simulink model "VCU_SW_1"  (R2023b)
settings: Solver=FixedStepDiscrete  StartTime=0.0  StopTime=inf  FixedStep=1e-2  RelTol=1e-3
PreLoadFcn:
  | RTWConfigurationCB('preloadfcn', bdroot);
InitFcn:
  | loadvar_ttc500
undefined symbols (not defined in the file): BrkPedalTypes, CabMovModeTypes, cFuseTempSensAcc_X, cFuseTempSensAcc_Y, cFuseTempSensVal_X, cFuseTempSensVal_Y, cTMSTempSensVal_X, cTMSTempSensVal_Y, cTransferCaseSpeedRatio, diag_state, DoorsPositionTypes, dP_filter_Y, DriverOccClassSystemTypes, ErrorValueTypes, fatal_error_callback, IO_ADC_NO_RANGE, LadderStatusTypes, pAnalogCabRotSensAcc, pAnalogCabRotSensMaxVolt, pAnalogCabRotSensMinVolt, pAnalogCabRotSensRange, pAnalogCabRotSensZeroVolt, pBrkActivePress, pCabTiltSensAcc, pCabTiltSensMaxCur, pCabTiltSensMinCur, pDistanceCorrection, pECANManual_BPNEnable, pECANManual_BPNEnabler_Flag, pFilterSensAccRes, pHDirMaxDiffFrq, pHDirSensHighLvl, pHDirSensLowLvl, pMainGearRatio, pMaxFilterSensRes, pMaxFirstPedalSensValue, pMaxFuseTempSensRes, pMaxPressLoss, pMaxPressSensCurrent, pMaxPressValue, pMaxPressValueHydMotAndPump, pMaxPressValueParkDrain, pMaxSecondPedalSensValue, pMaxTempSensVoltage, pMaxTempValue, pMaxTMSTempSensRes, pMinFilterSensRes, pMinFirstPedalSensValue, pMinFuseTempSensRes, pMinPressLoss, pMinPressSensCurrent, pMinPressValue, pMinSecondPedalSensValue, pMinTempSensVoltage, pMinTempValue, pMinTMSTempSensRes, pMotorRingTeethNum, pPedalSensAccuracyPct, pPedalSensAccuracyVolt, pPressLossTreshhold ... (+20)
libraries: TTlibrary x270, canmsglib x127, simulink x88
(part 6 of 19)

== system VCU_SW_1/InputLayer/Manual/GetManual/TSC1 ==
  CAN_ManualData_TSC1 : canmsglib/CAN Unpack  MsgList=(none)  MsgName=Man_TSC1  MsgIDType=Extended (29-bit identifier)  MsgIdentifier=402659111  MsgLength=8  SignalInfo={ 'Man_ContPurp', '35', '5', 'LE', 'unsigned', 'Standard', '0', '1', '0', '0', '31'; 'Man_EngOverContMode', '27', '2', 'LE', 'unsigned', 'Standard', '0', '1', '0', '0', '3'; 'Man_EngReqSpSl', '8', '16', 'LE', 'unsigned', 'Standard', '0', '0.125', '0', '0', '8191.875'; 'Man_EngReqTrqTL', '0', '8', 'LE', 'unsigned', 'Standard', '0', '1', '-125', '-125', '130'; 'Man_F_ContPurp', '40', '1', 'LE', 'unsigned', 'Standard', '0', '1', '0', '0', '1'; 'Man_F_EngOverContMode', '29', '1', 'LE', 'unsigned', 'Standard', '0', '1', '0', '0', '1'; 'Man_F_EngReqSpSl', '31', '1', 'LE', 'unsigned', 'Standard', '0', '1', '0', '0', '1'; 'Man_F_EngReqTrqTL', '30', '1', 'LE', 'unsigned', 'Standard', '0', '1', '0', '0', '1'; 'Man_F_OverContModePr', '34', '1', 'LE', 'unsigned', 'Standard', '0', '1', '0', '0', '1'; 'Man_F_ReqSpContCond', '26', '1', 'LE', 'unsigned', 'Standard', '0', '1', '0', '0', '1'; 'Man_OverContModePr', '32', '2', 'LE', 'unsigned', 'Standard', '0', '1', '0', '0', '3'; 'Man_ReqSpContCond', '24', '2', 'LE', 'unsigned', 'Standard', '0', '1', '0', '0', '3' }  IDPort=off  TimestampPort=off  ErrorPort=off  RemotePort=off  LengthPort=off  StatusPort=off  ApplyMinMax=off
  Data Store Write1 : DataStoreWrite  DataStoreName=ManualOutputInterfaceData  DataStoreElements=ManualOutputInterfaceData.TSC1_Man.Man_ContPurp#ManualOutputInterfaceData.TSC1_Man.Man_EngOverContMode#ManualOutputInterfaceData.TSC1_Man.Man_EngReqSpSl#ManualOutputInterfaceData.TSC1_Man.Man_EngReqTrqTL#ManualOutputInterfaceData.TSC1_Man.Man_F_ContPurp#ManualOutputInterfaceData.TSC1_Man.Man_F_EngOverContMode#ManualOutputInterfaceData.TSC1_Man.Man_F_EngReqSpSl#ManualOutputInterfaceData.TSC1_Man.Man_F_EngReqTrqTL#ManualOutputInterfaceData.TSC1_Man.Man_F_OverContModePr#ManualOutputInterfaceData.TSC1_Man.Man_F_ReqSpContCond#ManualOutputInterfaceData.TSC1_Man.Man_OverContModePr#ManualOutputInterfaceData.TSC1_Man.Man_ReqSpContCond  IndexOptions=Index vector (dialog)  Indices=1  OutputSizes=1
  Data Type Conversion : DataTypeConversion  OutDataTypeStr=int8  SaturateOnIntegerOverflow=off  RndMeth=Floor
  Terminator1 : Terminator
  read_message_ManualData_TSC1 : TTlibrary/CAN/read_message_name  channel=IO_CAN_CHANNEL_6  id_format=IO_CAN_EXT_FRAME  get_msg_info=off  message_names=there is no CAN Unpack blocks  message_info=|  id=402659111  ac_mask=536870911  retranslation=off  io_error=on  sample_time=-1
      | Message Name: Man_TSC1
      |  Message ID Type: Extended (29-bit identifier)
      |  Message ID: 402659111
      settings: SourceProductName=TT control 500 series
  wires:
  Data Type Conversion/1 -> Data Store Write1/4
  CAN_ManualData_TSC1/12 -> Data Store Write1/12
  CAN_ManualData_TSC1/11 -> Data Store Write1/11
  CAN_ManualData_TSC1/10 -> Data Store Write1/10
  CAN_ManualData_TSC1/9 -> Data Store Write1/9
  CAN_ManualData_TSC1/8 -> Data Store Write1/8
  CAN_ManualData_TSC1/7 -> Data Store Write1/7
  CAN_ManualData_TSC1/6 -> Data Store Write1/6
  CAN_ManualData_TSC1/5 -> Data Store Write1/5
  CAN_ManualData_TSC1/4 -> Data Type Conversion/1
  CAN_ManualData_TSC1/3 -> Data Store Write1/3
  CAN_ManualData_TSC1/2 -> Data Store Write1/2
  CAN_ManualData_TSC1/1 -> Data Store Write1/1
  read_message_ManualData_TSC1/2 -> Terminator1/1  "handler_err_402659111"
  read_message_ManualData_TSC1/1 -> CAN_ManualData_TSC1/1  "msg_402659111"

== system VCU_SW_1/InputLayer/Manual/GetManual/VLVCMD_HYD ==
  Data Store Write3 : DataStoreWrite  DataStoreName=ManualOutputInterfaceData  DataStoreElements=ManualOutputInterfaceData.VLVCMD_HYD.Man_Cab1LeftCylPortFlowCmdHyd#ManualOutputInterfaceData.VLVCMD_HYD.Man_Cab1LeftCylValveStateHyd#ManualOutputInterfaceData.VLVCMD_HYD.Man_Cab2RightCylFailSafeModeCmdHyd#ManualOutputInterfaceData.VLVCMD_HYD.Man_Cab2RightCylPortFlowCmdHyd#ManualOutputInterfaceData.VLVCMD_HYD.Man_Cab2RightCylValveStateHyd#ManualOutputInterfaceData.VLVCMD_HYD.Man_Cab1LeftCylFailSafeModeCmdHyd#ManualOutputInterfaceData.VLVCMD_HYD.Man_CabRotFailSafeModeCmdHyd#ManualOutputInterfaceData.VLVCMD_HYD.Man_CabRotPortFlowCmdHyd#ManualOutputInterfaceData.VLVCMD_HYD.Man_CabRotValveStateHyd#ManualOutputInterfaceData.VLVCMD_HYD.Man_F_Cab1LeftCylFailSafeModeCmdHyd#ManualOutputInterfaceData.VLVCMD_HYD.Man_F_Cab1LeftCylPortFlowCmdHyd#ManualOutputInterfaceData.VLVCMD_HYD.Man_F_Cab1LeftCylValveStateHyd#ManualOutputInterfaceData.VLVCMD_HYD.Man_F_Cab2RightCylFailSafeModeCmdHyd#ManualOutputInterfaceData.VLVCMD_HYD.Man_F_Cab2RightCylPortFlowCmdHyd#ManualOutputInterfaceData.VLVCMD_HYD.Man_F_Cab2RightCylValveStateHyd#ManualOutputInterfaceData.VLVCMD_HYD.Man_F_CabRotFailSafeModeCmdHyd#ManualOutputInterfaceData.VLVCMD_HYD.Man_F_CabRotPortFlowCmdHyd#ManualOutputInterfaceData.VLVCMD_HYD.Man_F_CabRotValveStateHyd  IndexOptions=Index vector (dialog)  Indices=1  OutputSizes=1
  Man_EEC2 : canmsglib/CAN Unpack  MsgList=(none)  MsgName=Man_VLVCMD_HYD  MsgIDType=Extended (29-bit identifier)  MsgIdentifier=402659879  MsgLength=8  SignalInfo={ 'Man_Cab1LeftCylPortFlowCmdHyd', '17', '8', 'LE', 'unsigned', 'Standard', '0', '0.4', '0', '0', '100'; 'Man_Cab1LeftCylValveStateHyd', '25', '4', 'LE', 'unsigned', 'Standard', '0', '1', '0', '0', '15'; 'Man_Cab2RightCylFailSafeModeCmd', '46', '2', 'LE', 'unsigned', 'Standard', '0', '1', '0', '0', '3'; 'Man_Cab2RightCylPortFlowCmdHyd', '34', '8', 'LE', 'unsigned', 'Standard', '0', '0.4', '0', '0', '100'; 'Man_Cab2RightCylValveStateHyd', '42', '4', 'LE', 'unsigned', 'Standard', '0', '1', '0', '0', '15'; 'Man_CabLeftCylFailSafeModeCmdHyd', '29', '2', 'LE', 'unsigned', 'Standard', '0', '1', '0', '0', '3'; 'Man_CabRotFailSafeModeCmdHyd', '12', '2', 'LE', 'unsigned', 'Standard', '0', '1', '0', '0', '3'; 'Man_CabRotPortFlowCmdHyd', '0', '8', 'LE', 'unsigned', 'Standard', '0', '0.4', '0', '0', '100'; 'Man_CabRotValveStateHyd', '8', '4', 'LE', 'unsigned', 'Standard', '0', '1', '0', '0', '15'; 'Man_F_Cab1LeftCylFailSafeModeCmd', '33', '1', 'LE', 'unsigned', 'Standard', '0', '1', '0', '0', '1'; 'Man_F_Cab1LeftCylPortFlowCmd', '31', '1', 'LE', 'unsigned', 'Standard', '0', '1', '0', '0', '1'; 'Man_F_Cab1LeftCylValveState', '32', '1', 'LE', 'unsigned', 'Standard', '0', '1', '0', '0', '1'; 'Man_F_Cab2RightCylFailSafeMode', '50', '1', 'LE', 'unsigned', 'Standard', '0', '1', '0', '0', '1'; 'Man_F_Cab2RightCylPortFlowCmd', '48', '1', 'LE', 'unsigned', 'Standard', '0', '1', '0', '0', '1'; 'Man_F_Cab2RightCylValveState', '49', '1', 'LE', 'unsigned', 'Standard', '0', '1', '0', '0', '1'; 'Man_F_CabRotFailSafeModeCmdHyd', '16', '1', 'LE', 'unsigned', 'Standard', '0', '1', '0', '0', '1'; 'Man_F_CabRotPortFlowCmdHyd', '14', '1', 'LE', 'unsigned', 'Standard', '0', '1', '0', '0', '1'; 'Man_F_CabRotValveStateHyd', '15', '1', 'LE', 'unsigned', 'Standard', '0', '1', '0', '0', '1' }  IDPort=off  TimestampPort=off  ErrorPort=off  RemotePort=off  LengthPort=off  StatusPort=off  ApplyMinMax=off
  Terminator1 : Terminator
  read_message_Man_EEC2 : TTlibrary/CAN/read_message_name  channel=IO_CAN_CHANNEL_6  id_format=IO_CAN_EXT_FRAME  get_msg_info=off  message_names=there is no CAN Unpack blocks  message_info=|  id=402660135  ac_mask=536870911  retranslation=off  io_error=on  sample_time=-1
      | Message Name: Man_TSC1
      |  Message ID Type: Extended (29-bit identifier)
      |  Message ID: 402659111
      settings: SourceProductName=TT control 500 series
  wires:
  read_message_Man_EEC2/1 -> Man_EEC2/1  "msg_402660135"
  Man_EEC2/17 -> Data Store Write3/17
  Man_EEC2/18 -> Data Store Write3/18
  Man_EEC2/14 -> Data Store Write3/14
  Man_EEC2/15 -> Data Store Write3/15
  Man_EEC2/12 -> Data Store Write3/12
  Man_EEC2/13 -> Data Store Write3/13
  Man_EEC2/16 -> Data Store Write3/16
  Man_EEC2/10 -> Data Store Write3/10
  Man_EEC2/9 -> Data Store Write3/9
  Man_EEC2/6 -> Data Store Write3/6
  read_message_Man_EEC2/2 -> Terminator1/1  "handler_err_402660135"
  Man_EEC2/7 -> Data Store Write3/7
  Man_EEC2/11 -> Data Store Write3/11
  Man_EEC2/8 -> Data Store Write3/8
  Man_EEC2/4 -> Data Store Write3/4
  Man_EEC2/2 -> Data Store Write3/2
  Man_EEC2/1 -> Data Store Write3/1
  Man_EEC2/3 -> Data Store Write3/3
  Man_EEC2/5 -> Data Store Write3/5

== system VCU_SW_1/InputLayer/Manual/GetManual/VLVCMD_STR ==
  CAN_ManualData_Params1 : canmsglib/CAN Unpack  MsgList=(none)  MsgName=Man_VLVCMD_STR  MsgIDType=Extended (29-bit identifier)  MsgIdentifier=402659623  MsgLength=8  SignalInfo={ 'Man_F_FailSafeModeCmdStr', '16', '1', 'LE', 'unsigned', 'Standard', '0', '1', '0', '0', '1'; 'Man_F_PortFlowCmdStr', '14', '1', 'LE', 'unsigned', 'Standard', '0', '1', '0', '0', '1'; 'Man_F_ValveStateStr', '15', '1', 'LE', 'unsigned', 'Standard', '0', '1', '0', '0', '1'; 'Man_FailSafeModeCmdStr', '12', '2', 'LE', 'unsigned', 'Standard', '0', '1', '0', '0', '3'; 'Man_PortFlowCmdStr', '0', '8', 'LE', 'unsigned', 'Standard', '0', '0.4', '0', '0', '100'; 'Man_ValveStateStr', '8', '4', 'LE', 'unsigned', 'Standard', '0', '1', '0', '0', '15' }  IDPort=off  TimestampPort=off  ErrorPort=off  RemotePort=off  LengthPort=off  StatusPort=off  ApplyMinMax=off
  Data Store Write2 : DataStoreWrite  DataStoreName=ManualOutputInterfaceData  DataStoreElements=ManualOutputInterfaceData.VLVCMD_STR.Man_F_FailSafeModeCmdStr#ManualOutputInterfaceData.VLVCMD_STR.Man_F_PortFlowCmdStr#ManualOutputInterfaceData.VLVCMD_STR.Man_F_ValveStateStr#ManualOutputInterfaceData.VLVCMD_STR.Man_FailSafeModeCmdStr#ManualOutputInterfaceData.VLVCMD_STR.Man_PortFlowCmdStr#ManualOutputInterfaceData.VLVCMD_STR.Man_ValveStateStr  IndexOptions=Index vector (dialog)  Indices=1  OutputSizes=1
  Terminator2 : Terminator
  read_message_ManualData_Params : TTlibrary/CAN/read_message_name  channel=IO_CAN_CHANNEL_6  id_format=IO_CAN_EXT_FRAME  get_msg_info=off  message_names=there is no CAN Unpack blocks  message_info=|  id=402659623  ac_mask=536870911  retranslation=off  io_error=on  sample_time=-1
      | Message Name: Man_Params
      |  Message ID Type: Extended (29-bit identifier)
      |  Message ID: 402658855
      settings: SourceProductName=TT control 500 series
  wires:
  CAN_ManualData_Params1/6 -> Data Store Write2/6
  CAN_ManualData_Params1/5 -> Data Store Write2/5
  CAN_ManualData_Params1/4 -> Data Store Write2/4
  CAN_ManualData_Params1/3 -> Data Store Write2/3
  CAN_ManualData_Params1/2 -> Data Store Write2/2
  CAN_ManualData_Params1/1 -> Data Store Write2/1
  read_message_ManualData_Params/2 -> Terminator2/1  "handler_err_402659623"
  read_message_ManualData_Params/1 -> CAN_ManualData_Params1/1  "msg_402659623"

== system VCU_SW_1/OutputLayer/OutputInterfaces/DigitalOutput1/SetDO1000msec ==
  function : TriggerPort  TriggerType=function-call  VariantControl=Variant
  Constant48 : Constant  Value=2  OutDataTypeStr=uint8
  Constant49 : Constant  OutDataTypeStr=uint8
  Data Store Read15 : DataStoreRead  DataStoreName=OutputInterfaceData  DataStoreElements=OutputInterfaceData.DO.lowBrakeFluidSensSupply  IndexOptions=Index vector (dialog)  Indices=1  OutputSizes=1
  Data Store Read61 : DataStoreRead  DataStoreName=ManualOutputInterfaceData  DataStoreElements=ManualOutputInterfaceData.DO_Man.man_lowBrakeFluidSensSupply  IndexOptions=Index vector (dialog)  Indices=1  OutputSizes=1
  Data Type Conversion25 : DataTypeConversion  OutDataTypeStr=boolean  SaturateOnIntegerOverflow=off  RndMeth=Floor
  Function Caller16 : FunctionCaller  FunctionPrototype=rawValue = convDIOStsTypeToNum(enumValue)  InputArgumentSpecifications=<Enter example>  OutputArgumentSpecifications=<Enter example>
  Logical Operator25 : Logic  Operator=OR  AllPortsSameDT=off  OutDataTypeStr=boolean
  Multiport Switch25 : MultiPortSwitch  DataPortOrder=Zero-based contiguous  Inputs=2  zeroidx=on  SaturateOnIntegerOverflow=off  InputSameDT=off
  Relational Operator50 : RelationalOperator  Operator===  OutDataTypeStr=boolean  RndMeth=Simplest  InputSameDT=off
  Relational Operator51 : RelationalOperator  Operator===  OutDataTypeStr=boolean  RndMeth=Simplest  InputSameDT=off
  Subsystem : Subsystem
  Terminator10 : Terminator
  setDigitalOutputValue16 : TTlibrary/DIO/setDigitalOutputValue  do_channel=IO_DO_41  diagnostic=FALSE  safety_conf=off  low_side_safety_channel=IO_DO_08  io_error=on  sample_time=-1
      settings: SourceProductName=TT control 500 series
  wires:
  Data Type Conversion25/1 -> Multiport Switch25/3
  Constant49/1 -> Relational Operator50/2
  Relational Operator50/1 -> Logical Operator25/2
  Multiport Switch25/1 -> setDigitalOutputValue16/1
  Logical Operator25/1 -> Multiport Switch25/1
  Data Store Read15/1 -> Function Caller16/1
  Relational Operator51/1 -> Logical Operator25/1
  Data Store Read61/1 -> Relational Operator51/1, Relational Operator50/1, Subsystem/1(In1)
  setDigitalOutputValue16/1 -> Terminator10/1
  Constant48/1 -> Relational Operator51/2
  Function Caller16/1 -> Multiport Switch25/2
  Subsystem/1(Out1) -> Data Type Conversion25/1

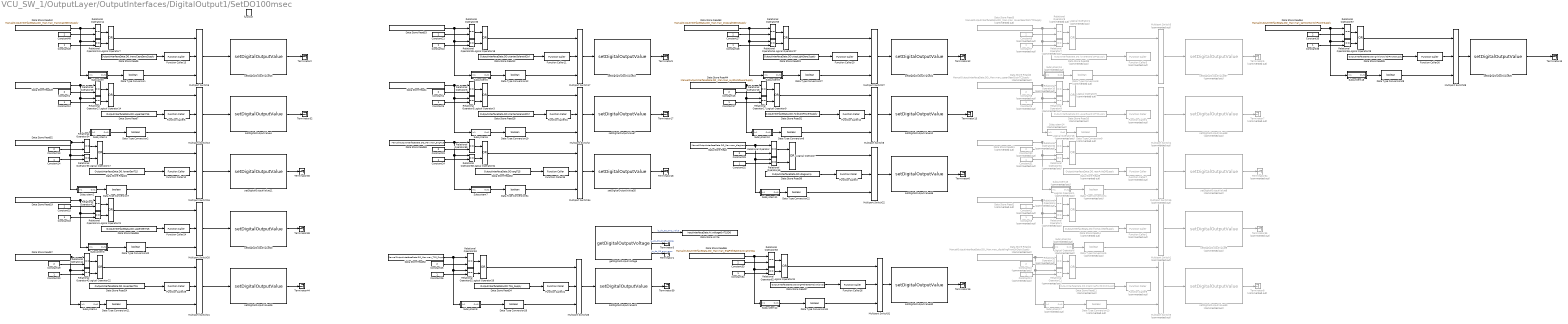
== system VCU_SW_1/OutputLayer/OutputInterfaces/DigitalOutput1/SetDO100msec ==
  function : TriggerPort  TriggerType=function-call  VariantControl=Variant
  Constant{1,4,13,15..16,19,21,23,25,27,29,33,35,48} (14 alike) : Constant  Value=2  OutDataTypeStr=uint8
  Constant{2,6,8,10,30} (5 alike) : Constant  Commented=on  Value=2  OutDataTypeStr=uint8
  Constant{3,7,9,11,31} (5 alike) : Constant  Commented=on  OutDataTypeStr=uint8
  Constant{5,12,14,17..18,20,22,24,26,28,32,34,36,49} (14 alike) : Constant  OutDataTypeStr=uint8
  Data Store Read : DataStoreRead  DataStoreName=ManualOutputInterfaceData  DataStoreElements=ManualOutputInterfaceData.DO_Man.man_diagLamp  IndexOptions=Index vector (dialog)  Indices=1  OutputSizes=1
  Data Store Read10 : DataStoreRead  Commented=on  DataStoreName=OutputInterfaceData  DataStoreElements=OutputInterfaceData.DO.upperGearDistrTCSupply  IndexOptions=Index vector (dialog)  Indices=1  OutputSizes=1
  Data Store Read11 : DataStoreRead  Commented=on  DataStoreName=OutputInterfaceData  DataStoreElements=OutputInterfaceData.DO.disablingFrontDrDistrSupply  IndexOptions=Index vector (dialog)  Indices=1  OutputSizes=1
  Data Store Read12 : DataStoreRead  DataStoreName=OutputInterfaceData  DataStoreElements=OutputInterfaceData.DO.starterSolenoidCtrl  IndexOptions=Index vector (dialog)  Indices=1  OutputSizes=1
  Data Store Read14 : DataStoreRead  Commented=on  DataStoreName=OutputInterfaceData  DataStoreElements=OutputInterfaceData.DO.frontAxleDifSupply  IndexOptions=Index vector (dialog)  Indices=1  OutputSizes=1
  Data Store Read19 : DataStoreRead  DataStoreName=ManualOutputInterfaceData  DataStoreElements=ManualOutputInterfaceData.DO_Man.man_upperGenT15  IndexOptions=Index vector (dialog)  Indices=1  OutputSizes=1
  Data Store Read2 : DataStoreRead  Commented=on  DataStoreName=ManualOutputInterfaceData  DataStoreElements=ManualOutputInterfaceData.DO_Man.man_frontAxleDifSupply  IndexOptions=Index vector (dialog)  Indices=1  OutputSizes=1
  Data Store Read22 : DataStoreRead  DataStoreName=OutputInterfaceData  DataStoreElements=OutputInterfaceData.DO.lowerGenT15  IndexOptions=Index vector (dialog)  Indices=1  OutputSizes=1
  Data Store Read23 : DataStoreRead  DataStoreName=OutputInterfaceData  DataStoreElements=OutputInterfaceData.DO.stopLightSensSupply  IndexOptions=Index vector (dialog)  Indices=1  OutputSizes=1
  Data Store Read24 : DataStoreRead  DataStoreName=OutputInterfaceData  DataStoreElements=OutputInterfaceData.DO.lowerGenT15  IndexOptions=Index vector (dialog)  Indices=1  OutputSizes=1
  Data Store Read27 : DataStoreRead  DataStoreName=OutputInterfaceData  DataStoreElements=OutputInterfaceData.DO.engPreheaterActivationSig  IndexOptions=Index vector (dialog)  Indices=1  OutputSizes=1
  Data Store Read28 : DataStoreRead  DataStoreName=OutputInterfaceData  DataStoreElements=OutputInterfaceData.DO.starterSolenoidCtrl  IndexOptions=Index vector (dialog)  Indices=1  OutputSizes=1
  Data Store Read3 : DataStoreRead  Commented=on  DataStoreName=ManualOutputInterfaceData  DataStoreElements=ManualOutputInterfaceData.DO_Man.man_lowerGearDistrTCSupply  IndexOptions=Index vector (dialog)  Indices=1  OutputSizes=1
  Data Store Read31 : DataStoreRead  DataStoreName=OutputInterfaceData  DataStoreElements=OutputInterfaceData.DO.HydCANPowerSupply  IndexOptions=Index vector (dialog)  Indices=1  OutputSizes=1
  Data Store Read32 : DataStoreRead  DataStoreName=OutputInterfaceData  DataStoreElements=OutputInterfaceData.DO.engT15  IndexOptions=Index vector (dialog)  Indices=1  OutputSizes=1
  Data Store Read34 : DataStoreRead  DataStoreName=OutputInterfaceData  DataStoreElements=OutputInterfaceData.DO.T15_Supply  IndexOptions=Index vector (dialog)  Indices=1  OutputSizes=1
  Data Store Read35 : DataStoreRead  DataStoreName=OutputInterfaceData  DataStoreElements=OutputInterfaceData.DO.IgnitionSwitchPowerSupply  IndexOptions=Index vector (dialog)  Indices=1  OutputSizes=1
  Data Store Read36 : DataStoreRead  DataStoreName=OutputInterfaceData  DataStoreElements=OutputInterfaceData.DO.diagLamp  IndexOptions=Index vector (dialog)  Indices=1  OutputSizes=1
  Data Store Read39 : DataStoreRead  Commented=on  DataStoreName=OutputInterfaceData  DataStoreElements=OutputInterfaceData.DO.lowerGearDistrTCSupply  IndexOptions=Index vector (dialog)  Indices=1  OutputSizes=1
  Data Store Read4 : DataStoreRead  DataStoreName=ManualOutputInterfaceData  DataStoreElements=ManualOutputInterfaceData.DO_Man.man_starterSolenoidCtrl  IndexOptions=Index vector (dialog)  Indices=1  OutputSizes=1
  Data Store Read40 : DataStoreRead  Commented=on  DataStoreName=ManualOutputInterfaceData  DataStoreElements=ManualOutputInterfaceData.DO_Man.man_upperGearDistrTCSupply  IndexOptions=Index vector (dialog)  Indices=1  OutputSizes=1
  Data Store Read41 : DataStoreRead  Commented=on  DataStoreName=ManualOutputInterfaceData  DataStoreElements=ManualOutputInterfaceData.DO_Man.man_disablingFrontDrDistrSupply  IndexOptions=Index vector (dialog)  Indices=1  OutputSizes=1
  Data Store Read42 : DataStoreRead  DataStoreName=ManualOutputInterfaceData  DataStoreElements=ManualOutputInterfaceData.DO_Man.man_transCaseSensSupply  IndexOptions=Index vector (dialog)  Indices=1  OutputSizes=1
  Data Store Read44 : DataStoreRead  DataStoreName=ManualOutputInterfaceData  DataStoreElements=ManualOutputInterfaceData.DO_Man.man_HydCANPowerSupply  IndexOptions=Index vector (dialog)  Indices=1  OutputSizes=1
  Data Store Read49 : DataStoreRead  DataStoreName=ManualOutputInterfaceData  DataStoreElements=ManualOutputInterfaceData.DO_Man.man_upperGenT15  IndexOptions=Index vector (dialog)  Indices=1  OutputSizes=1
  Data Store Read5 : DataStoreRead  DataStoreName=OutputInterfaceData  DataStoreElements=OutputInterfaceData.DO.transCaseSensSupply  IndexOptions=Index vector (dialog)  Indices=1  OutputSizes=1
  Data Store Read51 : DataStoreRead  Commented=on  DataStoreName=ManualOutputInterfaceData  DataStoreElements=ManualOutputInterfaceData.DO_Man.man_rearAxleDifSupply  IndexOptions=Index vector (dialog)  Indices=1  OutputSizes=1
  Data Store Read52 : DataStoreRead  DataStoreName=ManualOutputInterfaceData  DataStoreElements=ManualOutputInterfaceData.DO_Man.man_lowerGenT15  IndexOptions=Index vector (dialog)  Indices=1  OutputSizes=1
  Data Store Read53 : DataStoreRead  DataStoreName=ManualOutputInterfaceData  DataStoreElements=ManualOutputInterfaceData.DO_Man.man_starterSolenoidCtrl  IndexOptions=Index vector (dialog)  Indices=1  OutputSizes=1
  Data Store Read56 : DataStoreRead  DataStoreName=OutputInterfaceData  DataStoreElements=OutputInterfaceData.DO.upperGenT15  IndexOptions=Index vector (dialog)  Indices=1  OutputSizes=1
  Data Store Read57 : DataStoreRead  DataStoreName=ManualOutputInterfaceData  DataStoreElements=ManualOutputInterfaceData.DO_Man.man_lowerGenT15  IndexOptions=Index vector (dialog)  Indices=1  OutputSizes=1
  Data Store Read62 : DataStoreRead  DataStoreName=ManualOutputInterfaceData  DataStoreElements=ManualOutputInterfaceData.DO_Man.man_T15_Supply  IndexOptions=Index vector (dialog)  Indices=1  OutputSizes=1
  Data Store Read63 : DataStoreRead  DataStoreName=ManualOutputInterfaceData  DataStoreElements=ManualOutputInterfaceData.DO_Man.man_stopLightSensSupply  IndexOptions=Index vector (dialog)  Indices=1  OutputSizes=1
  Data Store Read64 : DataStoreRead  DataStoreName=ManualOutputInterfaceData  DataStoreElements=ManualOutputInterfaceData.DO_Man.man_IgnitionSwitchPowerSupply  IndexOptions=Index vector (dialog)  Indices=1  OutputSizes=1
  Data Store Read66 : DataStoreRead  DataStoreName=ManualOutputInterfaceData  DataStoreElements=ManualOutputInterfaceData.DO_Man.man_engPreheaterActivationSig  IndexOptions=Index vector (dialog)  Indices=1  OutputSizes=1
  Data Store Read69 : DataStoreRead  DataStoreName=ManualOutputInterfaceData  DataStoreElements=ManualOutputInterfaceData.DO_Man.man_engT15  IndexOptions=Index vector (dialog)  Indices=1  OutputSizes=1
  Data Store Read7 : DataStoreRead  DataStoreName=OutputInterfaceData  DataStoreElements=OutputInterfaceData.DO.upperGenT15  IndexOptions=Index vector (dialog)  Indices=1  OutputSizes=1
  Data Store Read9 : DataStoreRead  Commented=on  DataStoreName=OutputInterfaceData  DataStoreElements=OutputInterfaceData.DO.rearAxleDifSupply  IndexOptions=Index vector (dialog)  Indices=1  OutputSizes=1
  Data Store Write : DataStoreWrite  DataStoreName=InputInterfaceData  DataStoreElements=InputInterfaceData.AI.voltageOnT15DO  IndexOptions=Index vector (dialog)  Indices=1  OutputSizes=1
  Data Type Conversion{,2,6..7,12,19..22,26..28,31,34} (14 alike) : DataTypeConversion  OutDataTypeStr=boolean  SaturateOnIntegerOverflow=off  RndMeth=Floor
  Data Type Conversion{4..5,8..9,13} (5 alike) : DataTypeConversion  Commented=on  OutDataTypeStr=boolean  SaturateOnIntegerOverflow=off  RndMeth=Floor
  Function Caller{1,3..4,7,9} (5 alike) : FunctionCaller  Commented=on  FunctionPrototype=rawValue = convDIOStsTypeToNum(enumValue)  InputArgumentSpecifications=<Enter example>  OutputArgumentSpecifications=<Enter example>
  Function Caller{2,5,10..13,20..21,24,26,29..31,35} (14 alike) : FunctionCaller  FunctionPrototype=rawValue = convDIOStsTypeToNum(enumValue)  InputArgumentSpecifications=<Enter example>  OutputArgumentSpecifications=<Enter example>
  Logical Operator{,3,7,9,14,17..18,21..22,26..28,31,34} (14 alike) : Logic  Operator=OR  AllPortsSameDT=off  OutDataTypeStr=boolean
  Logical Operator{1,4..6,16} (5 alike) : Logic  Commented=on  Operator=OR  AllPortsSameDT=off  OutDataTypeStr=boolean
  Multiport Switch{1,3..5,15} (5 alike) : MultiPortSwitch  Commented=on  DataPortOrder=Zero-based contiguous  Inputs=2  zeroidx=on  SaturateOnIntegerOverflow=off  InputSameDT=off
  Multiport Switch{2,6,8,13,16..17,20..21,26..28,31,34} (13 alike) : MultiPortSwitch  DataPortOrder=Zero-based contiguous  Inputs=2  zeroidx=on  SaturateOnIntegerOverflow=off  InputSameDT=off
  Multiport Switch22 : MultiPortSwitch  DataPortOrder=Zero-based contiguous  Inputs=2  DiagnosticForDefault=None  zeroidx=on  SaturateOnIntegerOverflow=off  InputSameDT=off
  Relational Operator{,5..6,13..14,17..18,27..28,33..36,41..45,52..57,62..63,68..69} (28 alike) : RelationalOperator  Operator===  OutDataTypeStr=boolean  RndMeth=Simplest  InputSameDT=off
  Relational Operator{1,4,7..12,31..32} (10 alike) : RelationalOperator  Commented=on  Operator===  OutDataTypeStr=boolean  RndMeth=Simplest  InputSameDT=off
  Subsystem : Subsystem
  Subsystem1 : Subsystem
  Subsystem10 : Subsystem
  Subsystem11 : Subsystem
  Subsystem12 : Subsystem
  Subsystem13 : Subsystem  Commented=on
  Subsystem14 : Subsystem  Commented=on
  Subsystem15 : Subsystem  Commented=on
  Subsystem16 : Subsystem  Commented=on
  Subsystem17 : Subsystem  Commented=on
  Subsystem18 : Subsystem
  Subsystem2 : Subsystem
  Subsystem3 : Subsystem
  Subsystem4 : Subsystem
  Subsystem5 : Subsystem
  Subsystem6 : Subsystem
  Subsystem7 : Subsystem
  Subsystem8 : Subsystem
  Subsystem9 : Subsystem
  Terminator{1..3,6,9,13,16..17,32,36,38..39,42..44,48} (16 alike) : Terminator
  Terminator{5,7..8,34..35} (5 alike) : Terminator  Commented=on
  getDigitalOutputVoltage : TTlibrary/DIO/getDigitalOutputVoltage  do_channel=IO_DO_03  io_error=on  sample_time=-1
      settings: SourceProductName=TT control 500 series
  setDigitalOutputValue10 : TTlibrary/DIO/setDigitalOutputValue  do_channel=IO_DO_39  diagnostic=FALSE  safety_conf=off  low_side_safety_channel=IO_DO_08  io_error=on  sample_time=-1
      settings: SourceProductName=TT control 500 series
  setDigitalOutputValue11 : TTlibrary/DIO/setDigitalOutputValue  do_channel=IO_DO_20  diagnostic=FALSE  safety_conf=off  low_side_safety_channel=IO_DO_08  io_error=on  sample_time=-1
      settings: SourceProductName=TT control 500 series
  setDigitalOutputValue12 : TTlibrary/DIO/setDigitalOutputValue  do_channel=IO_DO_06  diagnostic=FALSE  safety_conf=off  low_side_safety_channel=IO_DO_08  io_error=on  sample_time=-1
      settings: SourceProductName=TT control 500 series
  setDigitalOutputValue13 : TTlibrary/DIO/setDigitalOutputValue  do_channel=IO_DO_45  diagnostic=FALSE  safety_conf=off  low_side_safety_channel=IO_DO_08  io_error=on  sample_time=-1
      settings: SourceProductName=TT control 500 series
  setDigitalOutputValue20 : TTlibrary/DIO/setDigitalOutputValue  do_channel=IO_DO_51  diagnostic=FALSE  safety_conf=off  low_side_safety_channel=IO_DO_08  io_error=on  sample_time=-1
      settings: SourceProductName=TT control 500 series
  setDigitalOutputValue21 : TTlibrary/DIO/setDigitalOutputValue  do_channel=IO_DO_03  diagnostic=FALSE  safety_conf=off  low_side_safety_channel=IO_DO_08  io_error=on  sample_time=-1
      settings: SourceProductName=TT control 500 series
  setDigitalOutputValue24 : TTlibrary/DIO/setDigitalOutputValue  do_channel=IO_DO_33  diagnostic=FALSE  safety_conf=off  low_side_safety_channel=IO_DO_08  io_error=on  sample_time=-1
      settings: SourceProductName=TT control 500 series
  setDigitalOutputValue25 : TTlibrary/DIO/setDigitalOutputValue  do_channel=IO_DO_07  diagnostic=FALSE  safety_conf=off  low_side_safety_channel=IO_DO_08  io_error=on  sample_time=-1
      settings: SourceProductName=TT control 500 series
  setDigitalOutputValue26 : TTlibrary/DIO/setDigitalOutputValue  do_channel=IO_DO_21  diagnostic=FALSE  safety_conf=off  low_side_safety_channel=IO_DO_08  io_error=on  sample_time=-1
      settings: SourceProductName=TT control 500 series
  setDigitalOutputValue30 : TTlibrary/DIO/setDigitalOutputValue  do_channel=IO_DO_24  diagnostic=FALSE  safety_conf=off  low_side_safety_channel=IO_DO_08  io_error=on  sample_time=-1
      settings: SourceProductName=TT control 500 series
  setDigitalOutputValue35 : TTlibrary/DIO/setDigitalOutputValue  do_channel=IO_DO_42  diagnostic=FALSE  safety_conf=off  low_side_safety_channel=IO_DO_08  io_error=on  sample_time=-1
      settings: SourceProductName=TT control 500 series
  setDigitalOutputValue36 : TTlibrary/DIO/setDigitalOutputValue  do_channel=IO_DO_34  diagnostic=FALSE  safety_conf=off  low_side_safety_channel=IO_DO_08  io_error=on  sample_time=-1
      settings: SourceProductName=TT control 500 series
  setDigitalOutputValue37 : TTlibrary/DIO/setDigitalOutputValue  Commented=on  do_channel=IO_DO_23  diagnostic=FALSE  safety_conf=off  low_side_safety_channel=IO_DO_08  io_error=on  sample_time=-1
      settings: SourceProductName=TT control 500 series
  setDigitalOutputValue38 : TTlibrary/DIO/setDigitalOutputValue  Commented=on  do_channel=IO_DO_37  diagnostic=FALSE  safety_conf=off  low_side_safety_channel=IO_DO_08  io_error=on  sample_time=-1
      settings: SourceProductName=TT control 500 series
  setDigitalOutputValue39 : TTlibrary/DIO/setDigitalOutputValue  Commented=on  do_channel=IO_DO_25  diagnostic=FALSE  safety_conf=off  low_side_safety_channel=IO_DO_08  io_error=on  sample_time=-1
      settings: SourceProductName=TT control 500 series
  setDigitalOutputValue4 : TTlibrary/DIO/setDigitalOutputValue  do_channel=IO_DO_50  diagnostic=FALSE  safety_conf=off  low_side_safety_channel=IO_DO_08  io_error=on  sample_time=-1
      settings: SourceProductName=TT control 500 series
  setDigitalOutputValue7 : TTlibrary/DIO/setDigitalOutputValue  do_channel=IO_DO_38  diagnostic=FALSE  safety_conf=off  low_side_safety_channel=IO_DO_08  io_error=on  sample_time=-1
      settings: SourceProductName=TT control 500 series
  setDigitalOutputValue8 : TTlibrary/DIO/setDigitalOutputValue  Commented=on  do_channel=IO_DO_18  diagnostic=FALSE  safety_conf=off  low_side_safety_channel=IO_DO_08  io_error=on  sample_time=-1
      settings: SourceProductName=TT control 500 series
  setDigitalOutputValue9 : TTlibrary/DIO/setDigitalOutputValue  Commented=on  do_channel=IO_DO_32  diagnostic=FALSE  safety_conf=off  low_side_safety_channel=IO_DO_08  io_error=on  sample_time=-1
      settings: SourceProductName=TT control 500 series
  wires:
  Logical Operator7/1 -> Multiport Switch6/1
  Multiport Switch6/1 -> setDigitalOutputValue13/1
  Function Caller13/1 -> Multiport Switch6/2
  Data Store Read5/1 -> Function Caller13/1
  Data Type Conversion/1 -> Multiport Switch6/3
  Relational Operator13/1 -> Logical Operator7/2
  setDigitalOutputValue13/1 -> Terminator2/1
  Data Store Read42/1 -> Relational Operator14/1, Relational Operator13/1, Subsystem/1(In1)
  Constant49/1 -> Relational Operator13/2
  Constant48/1 -> Relational Operator14/2
  Relational Operator14/1 -> Logical Operator7/1
  Function Caller5/1 -> Multiport Switch13/2
  Constant12/1 -> Relational Operator27/2
  setDigitalOutputValue4/1 -> Terminator32/1
  Data Store Read52/1 -> Relational Operator34/1, Relational Operator33/1, Subsystem2/1(In1)
  Relational Operator27/1 -> Logical Operator14/2
  Relational Operator34/1 -> Logical Operator17/1
  Constant13/1 -> Relational Operator34/2
  Constant1/1 -> Relational Operator28/2
  Relational Operator33/1 -> Logical Operator17/2
  Data Store Read49/1 -> Relational Operator28/1, Relational Operator27/1, Subsystem1/1(In1)
  Function Caller10/1 -> Multiport Switch16/2
  Logical Operator17/1 -> Multiport Switch16/1
  Data Store Read22/1 -> Function Caller10/1
  Relational Operator28/1 -> Logical Operator14/1
  Data Type Conversion7/1 -> Multiport Switch16/3
  Constant14/1 -> Relational Operator33/2
  Multiport Switch13/1 -> setDigitalOutputValue4/1
  Logical Operator14/1 -> Multiport Switch13/1
  setDigitalOutputValue11/1 -> Terminator36/1
  Data Store Read7/1 -> Function Caller5/1
  Multiport Switch16/1 -> setDigitalOutputValue11/1
  Data Type Conversion2/1 -> Multiport Switch13/3
  Constant15/1 -> Relational Operator42/2
  Logical Operator21/1 -> Multiport Switch20/1
  Relational Operator42/1 -> Logical Operator21/1
  Relational Operator41/1 -> Logical Operator21/2
  Constant18/1 -> Relational Operator41/2
  Data Store Read19/1 -> Relational Operator42/1, Relational Operator41/1, Subsystem3/1(In1)
  Multiport Switch20/1 -> setDigitalOutputValue20/1
  setDigitalOutputValue20/1 -> Terminator38/1
  Data Store Read56/1 -> Function Caller24/1
  Function Caller24/1 -> Multiport Switch20/2
  Data Type Conversion20/1 -> Multiport Switch20/3
  Relational Operator43/1 -> Logical Operator22/2
  Data Store Read24/1 -> Function Caller29/1
  Relational Operator44/1 -> Logical Operator22/1
  Multiport Switch21/1 -> setDigitalOutputValue26/1
  Data Type Conversion21/1 -> Multiport Switch21/3
  setDigitalOutputValue26/1 -> Terminator44/1
  Logical Operator22/1 -> Multiport Switch21/1
  Constant19/1 -> Relational Operator44/2
  Data Store Read57/1 -> Relational Operator44/1, Relational Operator43/1, Subsystem4/1(In1)
  Constant20/1 -> Relational Operator43/2
  Function Caller29/1 -> Multiport Switch21/2
  Data Store Read62/1 -> Relational Operator53/1, Relational Operator52/1, Subsystem8/1(In1)
  setDigitalOutputValue10/1 -> Terminator9/1
  Multiport Switch34/1 -> setDigitalOutputValue35/1
  Relational Operator36/1 -> Logical Operator18/1
  getDigitalOutputVoltage/3 -> Terminator1/1  "io_do_03_amp_error"
  Function Caller31/1 -> Multiport Switch2/2
  Data Type Conversion12/1 -> Multiport Switch17/3
  Data Store Read32/1 -> Function Caller35/1
  Logical Operator26/1 -> Multiport Switch26/1
  Multiport Switch17/1 -> setDigitalOutputValue10/1
  Data Store Read34/1 -> Function Caller21/1
  setDigitalOutputValue7/1 -> Terminator17/1
  Data Store Read12/1 -> Function Caller11/1
  Logical Operator34/1 -> Multiport Switch34/1
  Constant23/1 -> Relational Operator69/2
  Constant25/1 -> Relational Operator53/2
  Relational Operator5/1 -> Logical Operator3/2
  Function Caller11/1 -> Multiport Switch17/2
  Relational Operator52/1 -> Logical Operator26/2
  Constant26/1 -> Relational Operator52/2
  Relational Operator35/1 -> Logical Operator18/2
  Logical Operator18/1 -> Multiport Switch17/1
  getDigitalOutputVoltage/1 -> Data Store Write/1  "io_do_03_amp_value"
  setDigitalOutputValue21/1 -> Terminator39/1
  Relational Operator68/1 -> Logical Operator34/2
  Logical Operator3/1 -> Multiport Switch2/1
  Data Store Read69/1 -> Relational Operator69/1, Relational Operator68/1, Subsystem7/1(In1)
  Data Store Read4/1 -> Relational Operator6/1, Relational Operator5/1, Subsystem6/1(In1)
  Constant24/1 -> Relational Operator68/2
  Multiport Switch2/1 -> setDigitalOutputValue7/1
  getDigitalOutputVoltage/2 -> Terminator3/1  "io_do_03_amp_update"
  setDigitalOutputValue35/1 -> Terminator48/1
  Function Caller21/1 -> Multiport Switch26/2
  Data Type Conversion34/1 -> Multiport Switch34/3
  Data Store Read28/1 -> Function Caller31/1
  Multiport Switch26/1 -> setDigitalOutputValue21/1
  Relational Operator69/1 -> Logical Operator34/1
  Data Store Read53/1 -> Relational Operator36/1, Relational Operator35/1, Subsystem5/1(In1)
  Data Type Conversion26/1 -> Multiport Switch26/3
  Constant5/1 -> Relational Operator5/2
  Constant4/1 -> Relational Operator6/2
  Data Type Conversion19/1 -> Multiport Switch2/3
  Relational Operator6/1 -> Logical Operator3/1
  Constant22/1 -> Relational Operator35/2
  Constant21/1 -> Relational Operator36/2
  Relational Operator53/1 -> Logical Operator26/1
  Function Caller35/1 -> Multiport Switch34/2
  Function Caller20/1 -> Multiport Switch27/2
  Data Type Conversion27/1 -> Multiport Switch27/3
  Constant27/1 -> Relational Operator55/2
  Logical Operator27/1 -> Multiport Switch27/1
  Constant28/1 -> Relational Operator54/2
  Relational Operator55/1 -> Logical Operator27/1
  Multiport Switch27/1 -> setDigitalOutputValue24/1
  setDigitalOutputValue24/1 -> Terminator42/1
  Data Store Read63/1 -> Relational Operator55/1, Relational Operator54/1, Subsystem9/1(In1)
  Data Store Read23/1 -> Function Caller20/1
  Relational Operator54/1 -> Logical Operator27/2
  Data Store Read40/1 -> Relational Operator10/1, Relational Operator9/1, Subsystem14/1(In1)
  setDigitalOutputValue37/1 -> Terminator5/1
  Data Type Conversion8/1 -> Multiport Switch3/3
  Constant11/1 -> Relational Operator11/2
  Relational Operator1/1 -> Logical Operator1/2
  Constant10/1 -> Relational Operator12/2
  Relational Operator31/1 -> Logical Operator16/2
  Data Store Read51/1 -> Relational Operator32/1, Relational Operator31/1, Subsystem15/1(In1)
  Logical Operator6/1 -> Multiport Switch5/1
  Multiport Switch15/1 -> setDigitalOutputValue8/1
  setDigitalOutputValue8/1 -> Terminator34/1
  Relational Operator12/1 -> Logical Operator6/1
  setDigitalOutputValue9/1 -> Terminator35/1
  Logical Operator1/1 -> Multiport Switch1/1
  Constant3/1 -> Relational Operator1/2
  Multiport Switch5/1 -> setDigitalOutputValue39/1
  Constant31/1 -> Relational Operator31/2
  Logical Operator16/1 -> Multiport Switch15/1
  Data Store Read9/1 -> Function Caller7/1
  Relational Operator4/1 -> Logical Operator1/1
  Data Type Conversion4/1 -> Multiport Switch15/3
  Constant2/1 -> Relational Operator4/2
  Data Store Read14/1 -> Function Caller1/1
  Data Type Conversion13/1 -> Multiport Switch5/3
  Multiport Switch1/1 -> setDigitalOutputValue9/1
  setDigitalOutputValue39/1 -> Terminator8/1
  Relational Operator32/1 -> Logical Operator16/1
  Data Store Read3/1 -> Relational Operator8/1, Subsystem13/1(In1), Relational Operator7/1
  Relational Operator11/1 -> Logical Operator6/2
  Data Type Conversion5/1 -> Multiport Switch1/3
  Relational Operator7/1 -> Logical Operator4/2
  Data Store Read11/1 -> Function Caller9/1
  Constant6/1 -> Relational Operator8/2
  Constant30/1 -> Relational Operator32/2
  Multiport Switch4/1 -> setDigitalOutputValue38/1
  Data Store Read41/1 -> Relational Operator12/1, Relational Operator11/1, Subsystem17/1(In1)
  setDigitalOutputValue38/1 -> Terminator7/1
  Constant9/1 -> Relational Operator9/2
  Data Store Read10/1 -> Function Caller4/1
  Logical Operator5/1 -> Multiport Switch4/1
  Multiport Switch3/1 -> setDigitalOutputValue37/1
  Relational Operator10/1 -> Logical Operator5/1
  Data Type Conversion9/1 -> Multiport Switch4/3
  Logical Operator4/1 -> Multiport Switch3/1
  Data Store Read39/1 -> Function Caller3/1
  Relational Operator9/1 -> Logical Operator5/2
  Constant8/1 -> Relational Operator10/2
  Constant7/1 -> Relational Operator7/2
  Relational Operator8/1 -> Logical Operator4/1
  Data Store Read2/1 -> Relational Operator4/1, Relational Operator1/1, Subsystem16/1(In1)
  Relational Operator18/1 -> Logical Operator9/1
  Function Caller12/1 -> Multiport Switch8/2
  Data Store Read31/1 -> Function Caller12/1
  Logical Operator9/1 -> Multiport Switch8/1
  Constant17/1 -> Relational Operator17/2
  Constant16/1 -> Relational Operator18/2
  Relational Operator17/1 -> Logical Operator9/2
  setDigitalOutputValue12/1 -> Terminator13/1
  Data Type Conversion6/1 -> Multiport Switch8/3
  Data Store Read44/1 -> Relational Operator18/1, Relational Operator17/1, Subsystem10/1(In1)
  Multiport Switch8/1 -> setDigitalOutputValue12/1
  Data Store Read36/1 -> Function Caller2/1
  Data Store Read/1 -> Relational Operator/1, Relational Operator45/1, Subsystem11/1(In1)
  Relational Operator/1 -> Logical Operator/1
  Function Caller2/1 -> Multiport Switch22/2
  Constant29/1 -> Relational Operator/2
  setDigitalOutputValue36/1 -> Terminator6/1
  Multiport Switch22/1 -> setDigitalOutputValue36/1
  Relational Operator45/1 -> Logical Operator/2
  Logical Operator/1 -> Multiport Switch22/1
  Data Type Conversion22/1 -> Multiport Switch22/3
  Constant32/1 -> Relational Operator45/2
  Data Type Conversion31/1 -> Multiport Switch31/3
  setDigitalOutputValue30/1 -> Terminator16/1
  Function Caller26/1 -> Multiport Switch31/2
  Constant34/1 -> Relational Operator62/2
  Relational Operator63/1 -> Logical Operator31/1
  Logical Operator31/1 -> Multiport Switch31/1
  Multiport Switch31/1 -> setDigitalOutputValue30/1
  Relational Operator62/1 -> Logical Operator31/2
  Constant33/1 -> Relational Operator63/2
  Data Store Read66/1 -> Relational Operator63/1, Relational Operator62/1, Subsystem12/1(In1)
  Data Store Read27/1 -> Function Caller26/1
  Function Caller30/1 -> Multiport Switch28/2
  Logical Operator28/1 -> Multiport Switch28/1
  Relational Operator56/1 -> Logical Operator28/2
  Data Type Conversion28/1 -> Multiport Switch28/3
  Data Store Read35/1 -> Function Caller30/1
  Multiport Switch28/1 -> setDigitalOutputValue25/1
  Relational Operator57/1 -> Logical Operator28/1
  Constant35/1 -> Relational Operator57/2
  Constant36/1 -> Relational Operator56/2
  Data Store Read64/1 -> Relational Operator57/1, Relational Operator56/1, Subsystem18/1(In1)
  setDigitalOutputValue25/1 -> Terminator43/1
  Subsystem/1(Out1) -> Data Type Conversion/1
  Subsystem1/1(Out1) -> Data Type Conversion2/1
  Subsystem2/1(Out1) -> Data Type Conversion7/1
  Subsystem3/1(Out1) -> Data Type Conversion20/1
  Subsystem4/1(Out1) -> Data Type Conversion21/1
  Subsystem5/1(Out1) -> Data Type Conversion12/1
  Subsystem6/1(Out1) -> Data Type Conversion19/1
  Subsystem7/1(Out1) -> Data Type Conversion34/1
  Subsystem8/1(Out1) -> Data Type Conversion26/1
  Subsystem9/1(Out1) -> Data Type Conversion27/1
  Subsystem10/1(Out1) -> Data Type Conversion6/1
  Subsystem11/1(Out1) -> Data Type Conversion22/1
  Subsystem12/1(Out1) -> Data Type Conversion31/1
  Subsystem13/1(Out1) -> Data Type Conversion8/1
  Subsystem14/1(Out1) -> Data Type Conversion9/1
  Subsystem15/1(Out1) -> Data Type Conversion4/1
  Subsystem16/1(Out1) -> Data Type Conversion5/1
  Subsystem17/1(Out1) -> Data Type Conversion13/1
  Subsystem18/1(Out1) -> Data Type Conversion28/1
